simulink model "Controller_Tank1_Primitives"  (R2012b)
settings: Solver=FixedStepDiscrete  StartTime=0.0  StopTime=10.0  FixedStep=0.1  RelTol=1e-3
libraries: simulink x1
settings Model: Creator=Kerianne  LastModifiedBy=Kerianne
settings DataIOCC: SaveFormat=Structure
settings OptimizationCC: InlineParams=on

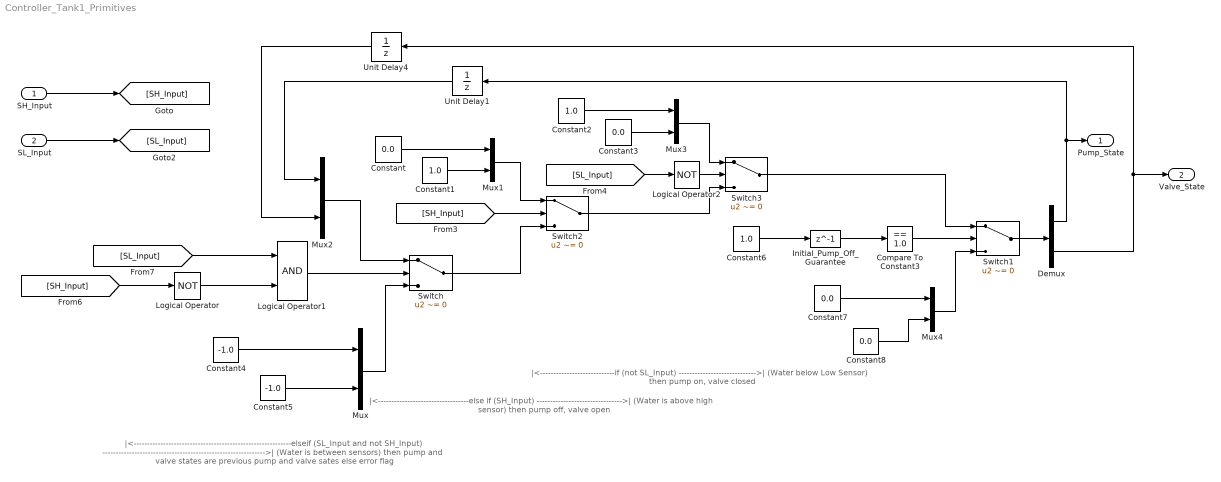
== system Controller_Tank1_Primitives ==
  note: |<----------------------------if (not SL_Input) ----------------------------->|
      | (Water below Low Sensor)
      | then pump on, valve closed
  note: |<----------------------------------else if (SH_Input) -------------------------------->|
      | (Water is above high sensor)
      | then pump off, valve open
  note: |<-----------------------------------------------------------elseif (SL_Input and not SH_Input) ------------------------------------------------------------->|
      | (Water is between sensors)
      | then pump and valve states are previous pump and valve sates
      | else error flag
  SH_Input : Inport
  SL_Input : Inport  Port=2  OutDataTypeStr=double
  Compare To Constant3 : simulink/Logic and Bit Operations/Compare To Constant  relop===  const=1.0  OutDataTypeStr=boolean
  Constant{,3,7..8} (4 alike) : Constant  Value=0.0
  Constant1 : Constant  Value=1.0
  Constant2 : Constant  Value=1.0
  Constant4 : Constant  Value=-1.0
  Constant5 : Constant  Value=-1.0
  Constant6 : Constant  Value=1.0
  Demux : Demux  Outputs=2
  Initial_Pump_Off_Guarantee : Delay  DelayLength=1
  Logical Operator : Logic  Operator=NOT  AllPortsSameDT=off  OutDataTypeStr=boolean
  Logical Operator1 : Logic  AllPortsSameDT=off  OutDataTypeStr=boolean
  Logical Operator2 : Logic  Operator=NOT  AllPortsSameDT=off  OutDataTypeStr=boolean
  Mux{,1..4} (5 alike) : Mux  Inputs=2
  Switch{,1..3} (4 alike) : Switch  Criteria=u2 ~= 0
  Unit Delay1 : UnitDelay  SampleTime=-1
  Unit Delay4 : UnitDelay  SampleTime=-1
  Pump_State : Outport
  Valve_State : Outport  Port=2
  wires:
  Mux/1 -> Switch/3
  Constant/1 -> Mux1/1
  Constant1/1 -> Mux1/2
  Unit Delay1/1 -> Mux2/1
  Mux2/1 -> Switch/1
  Logical Operator1/1 -> Switch/2
  [SL_Input] -> Logical Operator1/1
  Logical Operator/1 -> Logical Operator1/2
  [SH_Input] -> Logical Operator/1
  Switch/1 -> Switch2/3
  [SH_Input] -> Switch2/2
  Mux1/1 -> Switch2/1
  [SL_Input] -> Logical Operator2/1
  Constant2/1 -> Mux3/1
  Constant3/1 -> Mux3/2
  Mux3/1 -> Switch3/1
  SH_Input/1 -> [SH_Input]
  SL_Input/1 -> [SL_Input]
  Logical Operator2/1 -> Switch3/2
  Constant4/1 -> Mux/1
  Constant5/1 -> Mux/2
  Switch2/1 -> Switch3/3
  Constant6/1 -> Initial_Pump_Off_Guarantee/1
  Initial_Pump_Off_Guarantee/1 -> Compare To Constant3/1
  Compare To Constant3/1 -> Switch1/2
  Constant7/1 -> Mux4/1
  Constant8/1 -> Mux4/2
  Switch1/1 -> Demux/1
  Mux4/1 -> Switch1/3
  Switch3/1 -> Switch1/1
  Demux/1 -> Pump_State/1, Unit Delay1/1
  Demux/2 -> Valve_State/1, Unit Delay4/1
  Unit Delay4/1 -> Mux2/2
